simulink model "test_APS"  (R2022b)
settings: Solver=VariableStepAuto  StartTime=0.0  StopTime=2  RelTol=1e-3
undefined symbols (not defined in the file): raptor_xcp_function
libraries: Raptor_lib x8
settings Model: Creator=jackh  LastModifiedBy=jackh

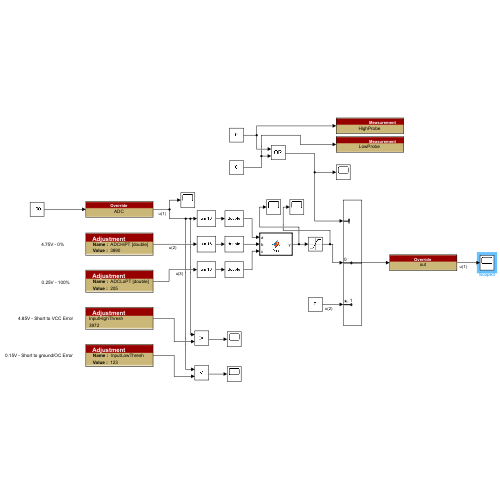
[thumbnail: Simulink's stored preview of the top-level diagram]
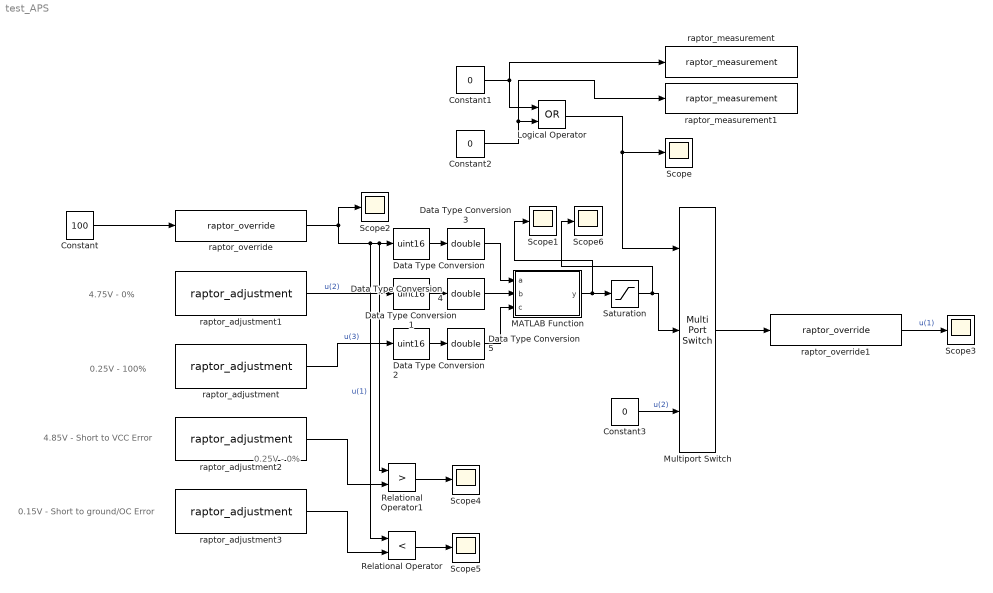
== system test_APS ==
  note: 0.25V - 100%
  note: 0.15V - Short to ground/OC Error
  note: 4.75V - 0%
  note: 4.85V - Short to VCC Error
  note: 0.25V - 0%
  Constant : Constant  Value=100
  Constant1 : Constant  Value=0
  Constant2 : Constant  Value=0
  Constant3 : Constant  Value=0
  Data Type Conversion : DataTypeConversion  OutDataTypeStr=uint16  SaturateOnIntegerOverflow=off  RndMeth=Floor
  Data Type Conversion1 : DataTypeConversion  OutDataTypeStr=uint16  SaturateOnIntegerOverflow=off  RndMeth=Floor
  Data Type Conversion2 : DataTypeConversion  OutDataTypeStr=uint16  SaturateOnIntegerOverflow=off  RndMeth=Floor
  Data Type Conversion3 : DataTypeConversion  OutDataTypeStr=double  SaturateOnIntegerOverflow=off  RndMeth=Floor
  Data Type Conversion4 : DataTypeConversion  OutDataTypeStr=double  SaturateOnIntegerOverflow=off  RndMeth=Floor
  Data Type Conversion5 : DataTypeConversion  OutDataTypeStr=double  SaturateOnIntegerOverflow=off  RndMeth=Floor
  Logical Operator : Logic  Operator=OR  AllPortsSameDT=off  OutDataTypeStr=boolean
  MATLAB Function : MATLAB Function  TreatAsAtomicUnit=on
  Multiport Switch : MultiPortSwitch  DataPortOrder=Zero-based contiguous  Inputs=2  zeroidx=on  SaturateOnIntegerOverflow=off  InputSameDT=off
  Relational Operator : RelationalOperator  Operator=<  OutDataTypeStr=boolean  RndMeth=Simplest  InputSameDT=off
  Relational Operator1 : RelationalOperator  Operator=>  OutDataTypeStr=boolean  RndMeth=Simplest  InputSameDT=off
  Saturation : Saturate  UpperLimit=100  LowerLimit=0
  Scope{,1..6} (7 alike) : Scope
  raptor_adjustment : Raptor_lib/Data Storage/raptor_adjustment  paramName=['ADCLoPT']  nameSource=Parameter  initValue=205  dataType=double  storage=Calibration  calDispType=Number  calEnum={'False', 'True'}  calGain=1.0  calOffset=0.0  calMax=inf  calMin=-inf  calFormat='-1'  calUnit='ADC'  calHelp="\"ADC Low Point\""  calAccess=1  calFunction=raptor_xcp_function(gcb)  calDispHeaders=off  calColHeaders={'Col1' 'Col2' 'Col3'}  calRowHeaders={'Row1' 'Row2' 'Row3'}
      settings: SourceProductName=Raptor
  raptor_adjustment1 : Raptor_lib/Data Storage/raptor_adjustment  paramName=['ADCHiPT']  nameSource=Parameter  initValue=3890  dataType=double  storage=Calibration  calDispType=Number  calEnum={'False', 'True'}  calGain=1.0  calOffset=0.0  calMax=inf  calMin=-inf  calFormat='-1'  calUnit='ADC'  calHelp="\"ADC High Point\""  calAccess=1  calFunction=raptor_xcp_function(gcb)  calDispHeaders=off  calColHeaders={'Col1' 'Col2' 'Col3'}  calRowHeaders={'Row1' 'Row2' 'Row3'}
      settings: SourceProductName=Raptor
  raptor_adjustment2 : Raptor_lib/Data Storage/raptor_adjustment  paramName=['InputHighThresh']  nameSource=Parameter  initValue=3972  dataType=double  storage=Calibration  calDispType=Number  calEnum={'False', 'True'}  calGain=1.0  calOffset=0.0  calMax=inf  calMin=-inf  calFormat='-1'  calUnit='ADC'  calHelp="\"Input out of range high point threshold\""  calAccess=1  calFunction=raptor_xcp_function(gcb)  calDispHeaders=off  calColHeaders={'Col1' 'Col2' 'Col3'}  calRowHeaders={'Row1' 'Row2' 'Row3'}
      settings: SourceProductName=Raptor
  raptor_adjustment3 : Raptor_lib/Data Storage/raptor_adjustment  paramName=['InputLowThresh']  nameSource=Parameter  initValue=123  dataType=double  storage=Calibration  calDispType=Number  calEnum={'False', 'True'}  calGain=1.0  calOffset=0.0  calMax=inf  calMin=-inf  calFormat='-1'  calUnit='ADC'  calHelp="\"Input out of range low point threshold\""  calAccess=1  calFunction=raptor_xcp_function(gcb)  calDispHeaders=off  calColHeaders={'Col1' 'Col2' 'Col3'}  calRowHeaders={'Row1' 'Row2' 'Row3'}
      settings: SourceProductName=Raptor
  raptor_measurement : Raptor_lib/Data Storage/raptor_measurement  paramName=['HighProbe']  nameSource=Parameter  calDispType=Number  calEnum={'False', 'True'}  calGain=1.0  calOffset=0.0  calMax=inf  calMin=-inf  calFormat='-1'  calUnit=''  calHelp=''  calAccess=1  calFunction=raptor_xcp_function(gcb)  calVisible=on
      settings: SourceProductName=Raptor
  raptor_measurement1 : Raptor_lib/Data Storage/raptor_measurement  paramName=['LowProbe']  nameSource=Parameter  calDispType=Number  calEnum={'False', 'True'}  calGain=1.0  calOffset=0.0  calMax=inf  calMin=-inf  calFormat='-1'  calUnit=''  calHelp=''  calAccess=1  calFunction=raptor_xcp_function(gcb)  calVisible=on
      settings: SourceProductName=Raptor
  raptor_override : Raptor_lib/Data Storage/raptor_override  paramName=['ADC']  nameSource=Parameter  measurement=Output  calDispType=Number  calEnum={'False', 'True'}  calGain=1.0  calOffset=0.0  calMax=inf  calMin=-inf  calFormat='-1'  calUnit=''  calHelp=''  calAccess=1  calFunction="[raptor_xcp_function(gcb) '|'  'Override']"
      settings: SourceProductName=Raptor
  raptor_override1 : Raptor_lib/Data Storage/raptor_override  paramName='out'  nameSource=Parameter  measurement=Output  calDispType=Number  calEnum={'False', 'True'}  calGain=1.0  calOffset=0.0  calMax=inf  calMin=-inf  calFormat='-1'  calUnit=''  calHelp=''  calAccess=1  calFunction="[raptor_xcp_function(gcb) '|'  'Override']"
      settings: SourceProductName=Raptor
  wires:
  Constant2/1 -> raptor_measurement1/1, Logical Operator/2
  Saturation/1 -> Scope6/1, Multiport Switch/2
  Data Type Conversion2/1 -> Data Type Conversion5/1
  Relational Operator/1 -> Scope5/1
  Data Type Conversion1/1 -> Data Type Conversion4/1
  Data Type Conversion/1 -> Data Type Conversion3/1
  Constant1/1 -> Logical Operator/1, raptor_measurement/1
  raptor_adjustment2/1 -> Relational Operator1/2
  Constant3/1 -> Multiport Switch/3  "u(2)"
  raptor_adjustment3/1 -> Relational Operator/2
  Relational Operator1/1 -> Scope4/1
  Logical Operator/1 -> Scope/1, Multiport Switch/1
  raptor_override/1 -> Scope2/1, Relational Operator/1, Data Type Conversion/1, Relational Operator1/1  "u(1)"
  Constant/1 -> raptor_override/1
  raptor_override1/1 -> Scope3/1  "u(1)"
  raptor_adjustment/1 -> Data Type Conversion2/1  "u(3)"
  raptor_adjustment1/1 -> Data Type Conversion1/1  "u(2)"
  Multiport Switch/1 -> raptor_override1/1
  MATLAB Function/1(y) -> Scope1/1, Saturation/1
  Data Type Conversion3/1 -> MATLAB Function/1(a)
  Data Type Conversion4/1 -> MATLAB Function/2(b)
  Data Type Conversion5/1 -> MATLAB Function/3(c)

== matlab function test_APS/MATLAB Function ==
  data: a input; y output; b input; c input
function y = fcn(a,b,c)
y = ((b-a)/(b-c))*100;
end
